simulink subsystem "subsys_dynamic_plaque_2021A"  (R2021a)
settings: Solver=VariableStepAuto  StartTime=0.0  StopTime=10.0  RelTol=1e-3
settings Model: Creator=antho  LastModifiedBy=alexi

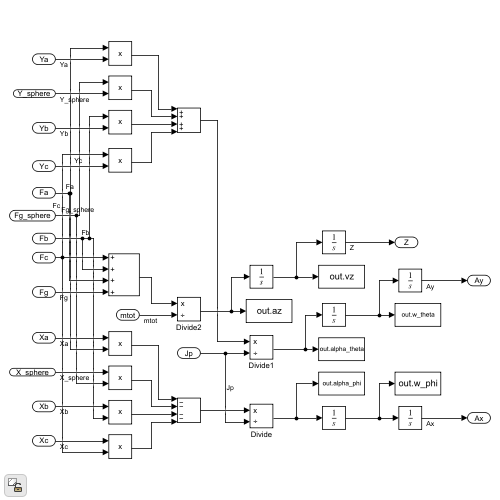
[thumbnail: Simulink's stored preview of the top-level diagram]
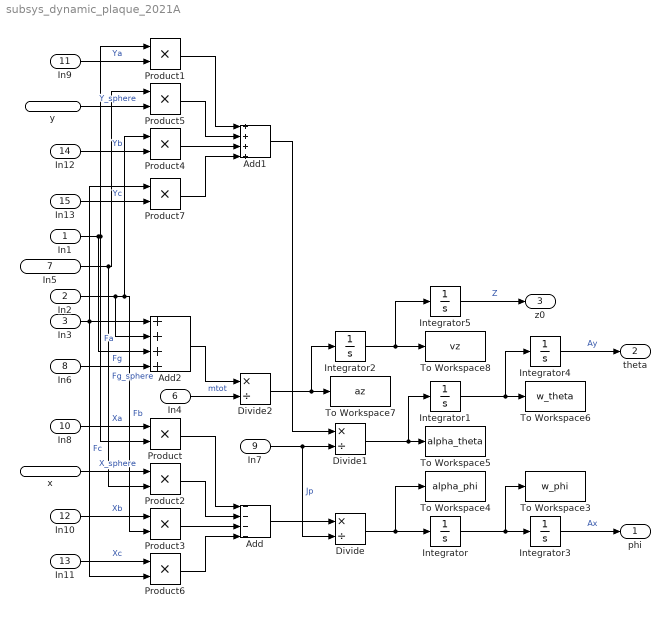
== system subsys_dynamic_plaque_2021A ==
  In1 : Inport
  In2 : Inport  Port=2
  In3 : Inport  Port=3
  x : Inport  Port=4
  y : Inport  Port=5
  In4 : Inport  Port=6
  In5 : Inport  Port=7
  In6 : Inport  Port=8
  In7 : Inport  Port=9
  In8 : Inport  Port=10
  In9 : Inport  Port=11
  In10 : Inport  Port=12
  In11 : Inport  Port=13
  In12 : Inport  Port=14
  In13 : Inport  Port=15
  Add : Sum  Inputs=----
  Add1 : Sum  Inputs=++++
  Add2 : Sum  Inputs=++++
  Divide : Product  Inputs=*/
  Divide1 : Product  Inputs=*/
  Divide2 : Product  Inputs=*/
  Integrator{,1..4} (5 alike) : Integrator
  Integrator5 : Integrator  InitialCondition=0.015
  Product{,1..7} (8 alike) : Product
  To Workspace3 : ToWorkspace  VariableName=w_phi  SaveFormat=Timeseries  SampleTime=-1
  To Workspace4 : ToWorkspace  VariableName=alpha_phi  SaveFormat=Timeseries  SampleTime=-1
  To Workspace5 : ToWorkspace  VariableName=alpha_theta  SaveFormat=Timeseries  SampleTime=-1
  To Workspace6 : ToWorkspace  VariableName=w_theta  SaveFormat=Timeseries  SampleTime=-1
  To Workspace7 : ToWorkspace  VariableName=az  SaveFormat=Timeseries  SampleTime=-1
  To Workspace8 : ToWorkspace  VariableName=vz  SaveFormat=Timeseries  SampleTime=-1
  phi : Outport
  theta : Outport  Port=2
  z0 : Outport  Port=3
  wires:
  y/1 -> Product5/2  "Y_sphere"
  Product7/1 -> Add1/4
  Add2/1 -> Divide2/1
  Divide/1 -> Integrator/1, To Workspace4/1
  Product5/1 -> Add1/2
  x/1 -> Product2/1  "X_sphere"
  Product2/1 -> Add/2
  In2/1 -> Product3/2, Product4/1, Add2/2  "Fb"
  In6/1 -> Add2/4  "Fg"
  Integrator4/1 -> theta/1  "Ay"
  In10/1 -> Product3/1  "Xb"
  Integrator5/1 -> z0/1  "Z"
  In4/1 -> Divide2/2  "mtot"
  Product1/1 -> Add1/1
  Product4/1 -> Add1/3
  Add/1 -> Divide/1
  Product6/1 -> Add/4
  In8/1 -> Product/1  "Xa"
  Integrator3/1 -> phi/1  "Ax"
  Integrator2/1 -> Integrator5/1, To Workspace8/1
  In9/1 -> Product1/2  "Ya"
  Add1/1 -> Divide1/1
  Product3/1 -> Add/3
  In13/1 -> Product7/2  "Yc"
  In11/1 -> Product6/1  "Xc"
  Divide1/1 -> Integrator1/1, To Workspace5/1
  Product/1 -> Add/1
  In7/1 -> Divide/2, Divide1/2  "Jp"
  In5/1 -> Product5/1, Product2/2  "Fg_sphere"
  In1/1 -> Product1/1, Product/2, Add2/3  "Fa"
  Integrator1/1 -> Integrator4/1, To Workspace6/1
  In3/1 -> Product7/1, Product6/2, Add2/1  "Fc"
  Divide2/1 -> Integrator2/1, To Workspace7/1
  Integrator/1 -> Integrator3/1, To Workspace3/1
  In12/1 -> Product4/2  "Yb"
